simulink model "uav_6dof_mvp"  (R2024b)
settings: Solver=VariableStepAuto  StartTime=0.0  StopTime=2  RelTol=1e-3
values from neighbouring files (symbols this model uses):
  m = z_wh/(b_w/2)    (= 0.106194690265)    [derivatives.m]    (also in main.m = 197.51552795; ngcp_plane.m = 1.08695652174)
undefined symbols (not defined in the file or in its folder): Ix, Iy, Iz
libraries: shared6dof x1
settings Model: Creator=natal  LastModifiedBy=natal

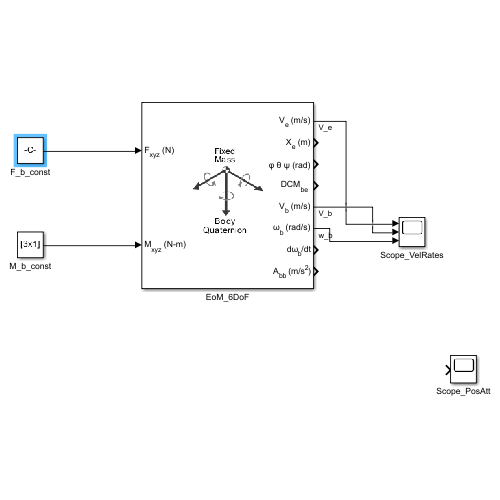
[thumbnail: Simulink's stored preview of the top-level diagram]
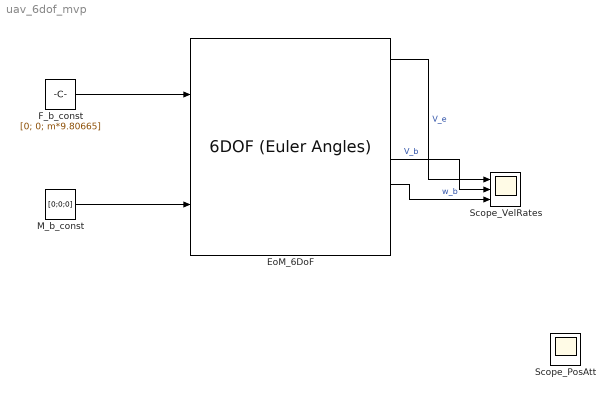
== system uav_6dof_mvp ==
  EoM_6DoF : shared6dof/6DOF (Euler Angles)  units=Metric (MKS)  mtype=Fixed  rep=Quaternion  xme_0=[0 0 0]  Vm_0=[25; 0; 0]  eul_0=[0 0 0]  pm_0=[0 0 0]  mass_0=m  mass_e=0.5  mass_f=2.0  inertia=[Ix 0 0; 0 Iy 0; 0 0 Iz]  inertia_e=eye(3)  inertia_f=2*eye(3)  k_quat=1.0  vre_flag=on  abi_flag=off  aMode=0  xme_statename=''  Vm_statename=''  eul_statename=''  quat_statename=''  pm_statename=''  mass_statename=''
      settings: LibrarySourceBlock=aerolib6dof2/6DOF (Quaternion)
  F_b_const : Constant  Value=[0; 0; m*9.80665]  VectorParams1D=off
  M_b_const : Constant  Value=[0;0;0]  VectorParams1D=off
  Scope_PosAtt : Scope
  Scope_VelRates : Scope  NumInputPorts=3
  wires:
  F_b_const/1 -> EoM_6DoF/1
  M_b_const/1 -> EoM_6DoF/2
  EoM_6DoF/1 -> Scope_VelRates/1  "V_e"
  EoM_6DoF/5 -> Scope_VelRates/2  "V_b"
  EoM_6DoF/6 -> Scope_VelRates/3  "w_b"
